simulink model "pblm1b"  (R2020b)
settings: Solver=VariableStepAuto  StartTime=0.0  StopTime=10.0  RelTol=1e-3
libraries: cstblocks x4
settings Model: Creator=Jonas  LastModifiedBy=Jonas

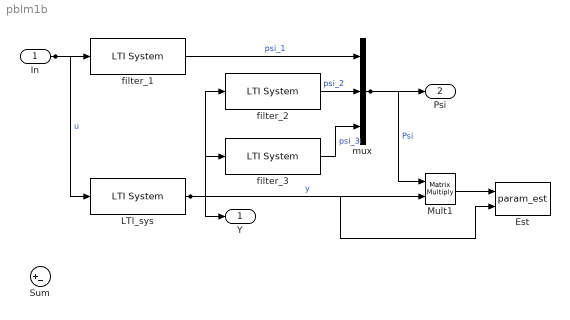
== system pblm1b ==
  In : Inport
  Est : M-S-Function  FunctionName=param_est
  LTI_sys : cstblocks/LTI System  sys=lti_sys  IC=x0
  Mult1 : Product  Inputs=**  Multiplication=Matrix(*)
  Sum : Sum  Inputs=|+-
  filter_1 : cstblocks/LTI System  sys=filter_1  IC=[]
  filter_2 : cstblocks/LTI System  sys=filter_2  IC=[]
  filter_3 : cstblocks/LTI System  sys=filter_3  IC=[]
  mux : Mux  Inputs=3
  Y : Outport
  Psi : Outport  Port=2
  wires:
  Mult1/1 -> Est/1
  In/1 -> LTI_sys/1, filter_1/1  "u"
  filter_3/1 -> mux/3  "psi_3"
  filter_2/1 -> mux/2  "psi_2"
  filter_1/1 -> mux/1  "psi_1"
  LTI_sys/1 -> filter_2/1, filter_3/1, Mult1/2, Y/1, Est/2  "y"
  mux/1 -> Mult1/1, Psi/1  "Psi"
